simulink model "MPC_RL_H2DF"  (R2023a)
settings: Solver=FixedStepAuto  StartTime=0.0  StopTime=inf  FixedStep=Ts  RelTol=1e-3
model workspace (MAT data in the model file):
  enable_IMEP_noise = 100
  enable_IMEP_offset = 1
values from neighbouring files (symbols this model uses):
  C2C_NMPC = init_C2C_NMPC_H2DF(C2C_NMPC.expdata)    [init_H2DFRL_GRU.m]
  LowerLimit = ([0.17e-3;350;-5;1e-3] - C2C_NMPC.Normalization.controls.mean)./(C2C_NMPC.Normalization.controls.std)    [init_H2DFRL_GRU.m]
  Ts = 0.08    [init_H2DFRL_GRU.m]
  UpperLimit = ([0.5e-3;900;2;5.5e-3] - C2C_NMPC.Normalization.controls.mean)./(C2C_NMPC.Normalization.controls.std)    [init_H2DFRL_GRU.m]
undefined symbols (not defined in the file or in its folder): CA50_offset, DiscIntNeverNeededParam, enable_CA50_noise, enable_CA50_offset, IMEP_offset
libraries: simulink x15, matrix_library x6, dspsigattribs x2, slctrlblks x2, statsLibrary x1, rllib x1
(part 1 of 4)
settings Model: Creator=norouziy  LastModifiedBy=vasu3
settings DebuggingCC: ParameterPrecisionLossMsg=none  UnconnectedInputMsg=warning  UnconnectedOutputMsg=warning  UnconnectedLineMsg=warning
settings ModelReferenceCC: EnableRefExpFcnMdlSchedulingChecks=on
settings RTWCC: DLArmComputeVersion=19.05

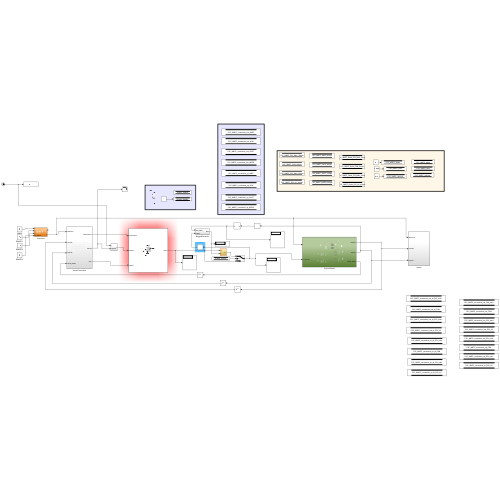
[thumbnail: Simulink's stored preview of the top-level diagram]
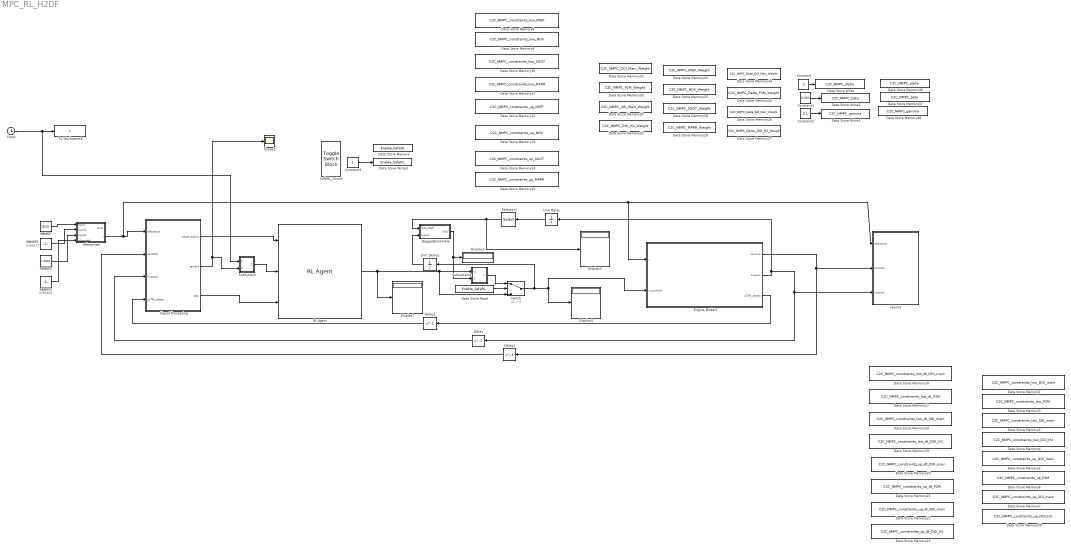
== system MPC_RL_H2DF ==
  BaggedEnsemble : Subsystem
  Clock : Clock
  Constant : Constant  Value=2
  Constant1 : Constant  Value=0.001
  Constant2 : Constant  Value=0.1
  Constant3 : Constant
  Data Store Memory : DataStoreMemory  DataStoreName=Enable_SafeRL  WriteAfterWriteMsg=warning  ShowAdditionalParam=off
  Data Store Memory1 : DataStoreMemory  DataStoreName=C2C_NMPC_constraints_low_DOI_main  WriteAfterWriteMsg=warning  ShowAdditionalParam=off
  Data Store Memory10 : DataStoreMemory  DataStoreName=C2C_NMPC_constraints_low_SOOT  WriteAfterWriteMsg=warning  ShowAdditionalParam=off
  Data Store Memory11 : DataStoreMemory  DataStoreName=C2C_NMPC_constraints_low_MPRR  WriteAfterWriteMsg=warning  ShowAdditionalParam=off
  Data Store Memory12 : DataStoreMemory  DataStoreName=C2C_NMPC_constraints_up_IMEP  WriteAfterWriteMsg=warning  ShowAdditionalParam=off
  Data Store Memory13 : DataStoreMemory  DataStoreName=C2C_NMPC_constraints_up_NOX  WriteAfterWriteMsg=warning  ShowAdditionalParam=off
  Data Store Memory14 : DataStoreMemory  DataStoreName=C2C_NMPC_constraints_up_SOOT  WriteAfterWriteMsg=warning  ShowAdditionalParam=off
  Data Store Memory15 : DataStoreMemory  DataStoreName=C2C_NMPC_constraints_up_MPRR  WriteAfterWriteMsg=warning  ShowAdditionalParam=off
  Data Store Memory16 : DataStoreMemory  DataStoreName=C2C_NMPC_constraints_low_dt_DOI_main  WriteAfterWriteMsg=warning  ShowAdditionalParam=off
  Data Store Memory17 : DataStoreMemory  DataStoreName=C2C_NMPC_constraints_low_dt_P2M  WriteAfterWriteMsg=warning  ShowAdditionalParam=off
  Data Store Memory18 : DataStoreMemory  DataStoreName=C2C_NMPC_constraints_low_dt_SOI_main  WriteAfterWriteMsg=warning  ShowAdditionalParam=off
  Data Store Memory19 : DataStoreMemory  DataStoreName=C2C_NMPC_constraints_low_dt_DOI_H2  WriteAfterWriteMsg=warning  ShowAdditionalParam=off
  Data Store Memory2 : DataStoreMemory  DataStoreName=C2C_NMPC_constraints_low_SOI_main  WriteAfterWriteMsg=warning  ShowAdditionalParam=off
  Data Store Memory20 : DataStoreMemory  DataStoreName=C2C_NMPC_constraints_up_dt_DOI_main  WriteAfterWriteMsg=warning  ShowAdditionalParam=off
  Data Store Memory21 : DataStoreMemory  DataStoreName=C2C_NMPC_constraints_up_dt_P2M  WriteAfterWriteMsg=warning  ShowAdditionalParam=off
  Data Store Memory22 : DataStoreMemory  DataStoreName=C2C_NMPC_constraints_up_dt_SOI_main  WriteAfterWriteMsg=warning  ShowAdditionalParam=off
  Data Store Memory23 : DataStoreMemory  DataStoreName=C2C_NMPC_constraints_up_dt_DOI_H1  WriteAfterWriteMsg=warning  ShowAdditionalParam=off
  Data Store Memory24 : DataStoreMemory  DataStoreName=C2C_NMPC_IMEP_Weight  WriteAfterWriteMsg=warning  ShowAdditionalParam=off
  Data Store Memory25 : DataStoreMemory  DataStoreName=C2C_NMPC_NOX_Weight  WriteAfterWriteMsg=warning  ShowAdditionalParam=off
  Data Store Memory26 : DataStoreMemory  DataStoreName=C2C_NMPC_Delta_SOI_Main_Weight  WriteAfterWriteMsg=warning  ShowAdditionalParam=off
  Data Store Memory27 : DataStoreMemory  DataStoreName=C2C_NMPC_Delta_DOI_H2_Weight  WriteAfterWriteMsg=warning  ShowAdditionalParam=off
  Data Store Memory28 : DataStoreMemory  DataStoreName=C2C_NMPC_SOOT_Weight  WriteAfterWriteMsg=warning  ShowAdditionalParam=off
  Data Store Memory29 : DataStoreMemory  DataStoreName=C2C_NMPC_MPRR_Weight  WriteAfterWriteMsg=warning  ShowAdditionalParam=off
  Data Store Memory3 : DataStoreMemory  DataStoreName=C2C_NMPC_constraints_low_P2M  WriteAfterWriteMsg=warning  ShowAdditionalParam=off
  Data Store Memory30 : DataStoreMemory  DataStoreName=C2C_NMPC_SOI_Main_Weight  WriteAfterWriteMsg=warning  ShowAdditionalParam=off
  Data Store Memory31 : DataStoreMemory  DataStoreName=C2C_NMPC_DOI_H2_Weight  WriteAfterWriteMsg=warning  ShowAdditionalParam=off
  Data Store Memory32 : DataStoreMemory  DataStoreName=C2C_NMPC_DOI_Main_Weight  WriteAfterWriteMsg=warning  ShowAdditionalParam=off
  Data Store Memory33 : DataStoreMemory  DataStoreName=C2C_NMPC_P2M_Weight  WriteAfterWriteMsg=warning  ShowAdditionalParam=off
  Data Store Memory34 : DataStoreMemory  DataStoreName=C2C_NMPC_Delta_DOI_Main_Weight  WriteAfterWriteMsg=warning  ShowAdditionalParam=off
  Data Store Memory35 : DataStoreMemory  DataStoreName=C2C_NMPC_Delta_P2M_Weight  WriteAfterWriteMsg=warning  ShowAdditionalParam=off
  Data Store Memory36 : DataStoreMemory  DataStoreName=C2C_NMPC_alpha  WriteAfterWriteMsg=warning  ShowAdditionalParam=off
  Data Store Memory37 : DataStoreMemory  DataStoreName=C2C_NMPC_beta  WriteAfterWriteMsg=warning  ShowAdditionalParam=off
  Data Store Memory38 : DataStoreMemory  DataStoreName=C2C_NMPC_gamma  WriteAfterWriteMsg=warning  ShowAdditionalParam=off
  Data Store Memory39 : DataStoreMemory  DataStoreName=C2C_NMPC_constraints_up_DOI_H2  WriteAfterWriteMsg=warning  ShowAdditionalParam=off
  Data Store Memory4 : DataStoreMemory  DataStoreName=C2C_NMPC_constraints_low_DOI_H2  WriteAfterWriteMsg=warning  ShowAdditionalParam=off
  Data Store Memory5 : DataStoreMemory  DataStoreName=C2C_NMPC_constraints_up_DOI_main  WriteAfterWriteMsg=warning  ShowAdditionalParam=off
  Data Store Memory6 : DataStoreMemory  DataStoreName=C2C_NMPC_constraints_up_P2M  WriteAfterWriteMsg=warning  ShowAdditionalParam=off
  Data Store Memory7 : DataStoreMemory  DataStoreName=C2C_NMPC_constraints_up_SOI_main  WriteAfterWriteMsg=warning  ShowAdditionalParam=off
  Data Store Memory8 : DataStoreMemory  DataStoreName=C2C_NMPC_constraints_low_IMEP  WriteAfterWriteMsg=warning  ShowAdditionalParam=off
  Data Store Memory9 : DataStoreMemory  DataStoreName=C2C_NMPC_constraints_low_NOX  WriteAfterWriteMsg=warning  ShowAdditionalParam=off
  Data Store Read : DataStoreRead  DataStoreName=Enable_SafeRL  IndexOptions=Index vector (dialog)  Indices=1  OutputSizes=1
  Data Store Write : DataStoreWrite  DataStoreName=C2C_NMPC_alpha  IndexOptions=Index vector (dialog)  Indices=1  OutputSizes=1
  Data Store Write1 : DataStoreWrite  DataStoreName=C2C_NMPC_beta  IndexOptions=Index vector (dialog)  Indices=1  OutputSizes=1
  Data Store Write2 : DataStoreWrite  DataStoreName=C2C_NMPC_gamma  IndexOptions=Index vector (dialog)  Indices=1  OutputSizes=1
  Data Store Write3 : DataStoreWrite  DataStoreName=Enable_SafeRL  IndexOptions=Index vector (dialog)  Indices=1  OutputSizes=1
  Delay : Delay  DelayLength=1  InitialCondition=rand(size(C2C_NMPC.xu0))
  Delay1 : Delay  DelayLength=1  InitialCondition=rand(8,1)
  Delay2 : Delay  DelayLength=1  InitialCondition=rand(size(C2C_NMPC.xu0))
  Display{1..4} (4 alike) : Display
  Engine Model2 : Subsystem
  RBMEP : Constant  Value=350220
  RBMEP1 : Constant  Value=0.56473
  RBMEP2 : Constant  Value=1.2601
  RBMEP3 : Constant  Value=0.95402
  RL Agent : rllib/RL Agent  Agent=saved_agent  ExternalActionAsInput=off  ProvideLastAction=off  ProvideCumRwd=off  TreatAsDirectFeedthrough=on  UseStrictObservationDataTypes=off
  SafeRL_Switch : ToggleSwitchBlock
      settings: Values={{'Off', 'On'}, [0 1]}
  Scope1 : Scope
  Selector1 : Selector  IndexOptions=Index vector (dialog)  Indices=[1]  OutputSizes=1
  Signal Processing : Subsystem
  Subsystem : Subsystem
  Subsystem1 : Subsystem
  Switch : Switch  Criteria=u2 > Threshold  SaturateOnIntegerOverflow=off  InputSameDT=off
  To Workspace8 : ToWorkspace  VariableName=t  SaveFormat=Timeseries  SampleTime=-1
  Unit Delay : UnitDelay  SampleTime=-1  HasFrameUpgradeWarning=on
  Unit Delay1 : UnitDelay  SampleTime=-1  HasFrameUpgradeWarning=on
  references : Subsystem
  results : Subsystem
  wires:
  Clock/1 -> Subsystem/1(In1), To Workspace8/1
  Signal Processing/2(reward) -> Scope1/1, Subsystem/2(reward)
  Signal Processing/3(stop) -> RL Agent/3
  Signal Processing/1(observations) -> RL Agent/1
  RBMEP/1 -> references/1(Input)
  references/2(r) -> Engine Model2/1(r), results/1(reference), Signal Processing/1(reference)
  Delay/1 -> Signal Processing/3(Outputs)
  Constant2/1 -> Data Store Write2/1
  Constant1/1 -> Data Store Write1/1
  Constant/1 -> Data Store Write/1
  Delay1/1 -> Signal Processing/4(LSTM_states)
  RBMEP1/1 -> references/2(Input1)
  RBMEP2/1 -> references/3(Input2)
  Subsystem/1(Out1) -> RL Agent/2
  Delay2/1 -> Signal Processing/2(controls)
  Engine Model2/1(controls) -> Delay2/1, results/2(controls)
  Engine Model2/2(outputs) -> Unit Delay/1, Delay/1, results/3(outputs)
  Engine Model2/3(LSTM_states) -> Delay1/1
  BaggedEnsemble/1(NOx) -> Subsystem1/2(In1), Display2/1
  RL Agent/1 -> Subsystem1/1(u1), Switch/3, Display1/1
  Unit Delay/1 -> Selector1/1
  Selector1/1 -> BaggedEnsemble/1(last_IMEP), Display3/1
  Subsystem1/1(u*1) -> Switch/1
  RBMEP3/1 -> references/4(rchange4)
  Data Store Read/1 -> Switch/2
  Switch/1 -> Unit Delay1/1, Engine Model2/2(rl_controls), Display4/1
  Constant3/1 -> Data Store Write3/1
  Unit Delay1/1 -> BaggedEnsemble/2(Inputs)

== system MPC_RL_H2DF/BaggedEnsemble ==
  last_IMEP : Inport
  Inputs : Inport  Port=2
  Mux : Mux  Inputs=2
  RegressionEnsemble Predict : statsLibrary/Regression/RegressionEnsemble Predict  TrainedLearner=trainedModel.RegressionEnsemble  OutMin=[]  OutMax=[]  WeakLearnerOutMin=[]  WeakLearnerOutMax=[]
  NOx : Outport
  wires:
  Mux/1 -> RegressionEnsemble Predict/1
  RegressionEnsemble Predict/1 -> NOx/1
  Inputs/1 -> Mux/1
  last_IMEP/1 -> Mux/2

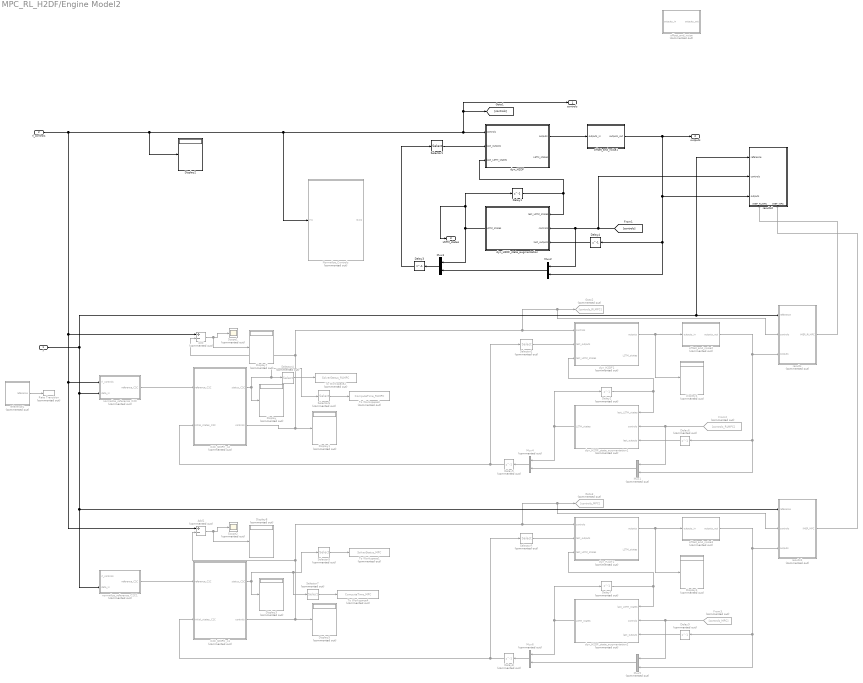
== system MPC_RL_H2DF/Engine Model2 ==
  r : Inport
  rl_controls : Inport  Port=2
  Add : Sum  Commented=on  Inputs=+-
  Add1 : Sum  Commented=on  Inputs=+-
  C2C_NMPC_n1 : Subsystem  Commented=on  VariantControl=C2C_NMPC_n2
  C2C_NMPC_n2 : Subsystem  Commented=on  VariantControl=C2C_NMPC_n2
  Delay1 : Delay  DelayLength=1  InitialCondition=C2C_NMPC.x0(1:C2C_NMPC.Dims.n_LSTM_states)
  Delay2 : Delay  Commented=on  DelayLength=1  InitialCondition=C2C_NMPC.x0(1:C2C_NMPC.Dims.n_LSTM_states)
  Delay3 : Delay  DelayLength=1  InitialCondition=C2C_NMPC.x0
  Delay4 : Delay  DelayLength=1  InitialCondition=C2C_NMPC.x0((C2C_NMPC.Dims.n_states - C2C_NMPC.Dims.n_outputs + 1):C2C_NMPC.Dims.n_states)
  Delay5 : Delay  Commented=on  DelayLength=1  InitialCondition=C2C_NMPC.x0
  Delay6 : Delay  Commented=on  DelayLength=1  InitialCondition=C2C_NMPC.x0((C2C_NMPC.Dims.n_states - C2C_NMPC.Dims.n_outputs + 1):C2C_NMPC.Dims.n_states)
  Delay7 : Delay  Commented=on  DelayLength=1  InitialCondition=C2C_NMPC.x0(1:C2C_NMPC.Dims.n_LSTM_states)
  Delay8 : Delay  Commented=on  DelayLength=1  InitialCondition=C2C_NMPC.x0
  Delay9 : Delay  Commented=on  DelayLength=1  InitialCondition=C2C_NMPC.x0((C2C_NMPC.Dims.n_states - C2C_NMPC.Dims.n_outputs + 1):C2C_NMPC.Dims.n_states)
  Display{,1,3..8} (8 alike) : Display  Commented=on
  Display2 : Display
  From2 : From  Commented=on  GotoTag=controls_RLMPC
  From3 : From  Commented=on  GotoTag=controls_MPC
  Goto2 : Goto  Commented=on  GotoTag=controls_RLMPC
  Goto3 : Goto  Commented=on  GotoTag=controls_MPC
  Mux{1,4..6} (4 alike) : Mux  Commented=on  Inputs=2
  Mux2 : Mux  Inputs=2
  Mux3 : Mux  Inputs=2
  Normalise_Controls : Subsystem  Commented=on
  Rate Transition : RateTransition  Commented=on  Integrity=off  OutPortSampleTime=Ts
  Scope1 : Scope  Commented=on
  Scope2 : Scope  Commented=on
  Selector1 : Selector  IndexOptions=Index vector (dialog)  Indices=[(C2C_NMPC.Dims.n_states - C2C_NMPC.Dims.n_outputs + 1):C2C_NMPC.Dims.n_states]  OutputSizes=1
  Selector2 : Selector  Commented=on  IndexOptions=Index vector (dialog)  Indices=[(C2C_NMPC.Dims.n_states - C2C_NMPC.Dims.n_outputs + 1):C2C_NMPC.Dims.n_states]  OutputSizes=1
  Selector3 : Selector  Commented=on  IndexOptions=Index vector (dialog)  Indices=[(C2C_NMPC.Dims.n_states - C2C_NMPC.Dims.n_outputs + 1):C2C_NMPC.Dims.n_states]  OutputSizes=1
  Selector4 : Selector  Commented=on  IndexOptions=Index vector (dialog)  Indices=1  OutputSizes=1
  Selector5 : Selector  Commented=on  IndexOptions=Index vector (dialog)  Indices=1  OutputSizes=1
  Selector6 : Selector  Commented=on  IndexOptions=Index vector (dialog)  Indices=3  OutputSizes=1
  Selector7 : Selector  Commented=on  IndexOptions=Index vector (dialog)  Indices=3  OutputSizes=1
  To Workspace1 : ToWorkspace  Commented=on  VariableName=SolverStatus_MPC  SampleTime=-1
  To Workspace2 : ToWorkspace  Commented=on  VariableName=SolverStatus_RLMPC  SampleTime=-1
  To Workspace3 : ToWorkspace  Commented=on  VariableName=ComputeTime_RLMPC  SampleTime=-1
  To Workspace4 : ToWorkspace  Commented=on  VariableName=ComputeTime_MPC  SampleTime=-1
  dyn_H2DF : Subsystem
  dyn_H2DF1 : Subsystem  Commented=on
  dyn_H2DF2 : Subsystem  Commented=on
  dyn_H2DF_state_augmentation : Subsystem
  dyn_H2DF_state_augmentation1 : Subsystem  Commented=on
  dyn_H2DF_state_augmentation2 : Subsystem  Commented=on
  normalize_reference_C2C : Subsystem  Commented=on
  normalize_reference_C2C1 : Subsystem  Commented=on
  offset_and_noise : Subsystem  Commented=on
  offset_and_noise1 : Subsystem
  offset_and_noise2 : Subsystem  Commented=on
  offset_and_noise3 : Subsystem  Commented=on
  reference1 : Subsystem  Commented=on
  results : Subsystem  Commented=on
  results1 : Subsystem  Commented=on
  results2 : Subsystem
      settings: PortSchema="{\"entries\":[{\"content\":{\"sides\":[{\"content\":{\"connectorIds\":[\"In1\",\"In2\",\"In3\"]},\"type\":\"ConnectorPlacement.EquallySpacedRectSide\",\"uuid\":\"75c69b80-8417-4b18-a9f8-39f8bddf459c\"},{\"content\":{\"side\":\"RIGHT\"},\"type\":\"ConnectorPlacement.EquallySpacedRectSide\",\"uuid\":\"4217b16a-0e70-4cec-a2f5-17ebe6dd1f5c\"},{\"content\":{\"side\":\"TOP\"},\"type\":\"ConnectorPlacement.EquallySpacedRectSide\",\"uuid\":\"1a4bc296-7285-4f1a-9d1a-4ffa534b2784\"},{\"content\":{\"connectorIds\":[\"In4\",\"In5\"],\"side\":\"BOTTOM\"},\"type\":\"ConnectorPlacement.EquallySpacedRectSide\",\"uuid\":\"31d565b7-d93d-4aac-b998-bcfa263f4420\"}]},\"type\":\"ConnectorPlacement.EquallySpacedConnector\",\"uuid\":\"a3bd06e2-48d8-47a5-9635-2e0335e011af\"}],\"packageUris\":[\"http://schema.mathworks.com/mf0/Connector/R2020b\"],\"version\":\"1.0\"}"
  controls : Outport
  outputs : Outport  Port=2
  LSTM_states : Outport  Port=3
  wires:
  Mux3/1 -> Delay3/1
  Delay1/1 -> dyn_H2DF/3(last_LSTM_states), dyn_H2DF_state_augmentation/1(last_LSTM_states)
  [controls] -> results2/2(controls), dyn_H2DF_state_augmentation/2(controls), Mux2/1
  Delay3/1 -> Selector1/1
  Delay4/1 -> dyn_H2DF_state_augmentation/3(last_outputs)
  Mux2/1 -> Mux3/2
  Selector1/1 -> dyn_H2DF/2(last_outputs)
  dyn_H2DF/1(outputs) -> offset_and_noise1/1(outputs_in)
  dyn_H2DF_state_augmentation/1(LSTM_states) -> LSTM_states/1, Delay1/1, Mux3/1
  offset_and_noise1/1(outputs_out) -> results2/3(outputs), Delay4/1, Mux2/2, outputs/1
  normalize_reference_C2C/1(reference_C2C) -> C2C_NMPC_n2/1(reference_C2C)
  C2C_NMPC_n2/2(controls) -> Add/2, results/2(controls), Goto2/1, dyn_H2DF1/1(controls), Display1/1
  reference1/1(reference) -> Rate Transition/1
  Delay6/1 -> dyn_H2DF_state_augmentation1/3(last_outputs)
  C2C_NMPC_n2/1(status_C2C) -> Selector6/1, Selector4/1, Display/1
  Mux1/1 -> Mux4/2
  dyn_H2DF_state_augmentation1/1(LSTM_states) -> Delay2/1, Mux4/1
  From2/1 -> dyn_H2DF_state_augmentation1/2(controls), Mux1/1
  dyn_H2DF1/1(outputs) -> Display4/1, offset_and_noise2/1(outputs_in)
  Mux4/1 -> Delay5/1
  Selector2/1 -> dyn_H2DF1/2(last_outputs)
  Delay5/1 -> C2C_NMPC_n2/2(initial_states_C2C), Selector2/1
  Delay2/1 -> dyn_H2DF1/3(last_LSTM_states), dyn_H2DF_state_augmentation1/1(last_LSTM_states)
  Add/1 -> Display7/1, Scope1/1
  offset_and_noise2/1(outputs_out) -> results/3(outputs), Delay6/1, Mux1/2
  normalize_reference_C2C1/1(reference_C2C) -> C2C_NMPC_n1/1(reference_C2C)
  Mux5/1 -> Mux6/2
  Mux6/1 -> Delay8/1
  dyn_H2DF2/1(outputs) -> Display6/1, offset_and_noise3/1(outputs_in)
  From3/1 -> dyn_H2DF_state_augmentation2/2(controls), Mux5/1
  offset_and_noise3/1(outputs_out) -> results1/3(outputs), Delay9/1, Mux5/2
  C2C_NMPC_n1/2(controls) -> results1/2(controls), Goto3/1, dyn_H2DF2/1(controls), Add1/2, Display5/1
  Delay7/1 -> dyn_H2DF2/3(last_LSTM_states), dyn_H2DF_state_augmentation2/1(last_LSTM_states)
  Add1/1 -> Display8/1, Scope2/1
  Delay9/1 -> dyn_H2DF_state_augmentation2/3(last_outputs)
  Delay8/1 -> C2C_NMPC_n1/2(initial_states_C2C), Selector3/1
  Selector3/1 -> dyn_H2DF2/2(last_outputs)
  dyn_H2DF_state_augmentation2/1(LSTM_states) -> Delay7/1, Mux6/1
  rl_controls/1 -> Display2/1, Normalise_Controls/1(In1), controls/1, [controls], dyn_H2DF/1(controls), Add1/1, normalize_reference_C2C/1(rl_controls), Add/1
  r/1 -> results1/1(reference), normalize_reference_C2C1/2(data_in), normalize_reference_C2C/2(data_in), results2/1(reference), results/1(reference)
  results/1(IMEP_RLMPC) -> results2/4(IMEP_RLMPC)
  results1/1(IMEP_MPC) -> results2/5(IMEP_MPC)
  Selector4/1 -> To Workspace2/1
  Selector5/1 -> To Workspace1/1
  Selector6/1 -> To Workspace3/1
  Selector7/1 -> To Workspace4/1
  C2C_NMPC_n1/1(status_C2C) -> Display3/1, Selector7/1, Selector5/1

== system MPC_RL_H2DF/Signal Processing ==
  reference : Inport
  controls : Inport  Port=2
  Outputs : Inport  Port=3
  LSTM_states : Inport  Port=4
  Normalization : Subsystem  Commented=on
  calculate reward : Subsystem
  generate observations1 : Subsystem
  stop simulation : Subsystem
  observations : Outport
  reward : Outport  Port=2
  stop : Outport  Port=3
  wires:
  calculate reward/1(reward) -> reward/1
  stop simulation/1(stop) -> stop/1
  generate observations1/1(observations) -> observations/1
  reference/1 -> generate observations1/2(Reference), calculate reward/1(Reference)
  Outputs/1 -> stop simulation/1(Output), calculate reward/3(outputs), generate observations1/1(Outputs)
  controls/1 -> calculate reward/2(controls)
  LSTM_states/1 -> generate observations1/3(LSTM States)

== system MPC_RL_H2DF/Subsystem ==
  In1 : Inport
  reward : Inport  Port=2
  If : If  IfExpression=u1 > 0.08
  If Action Subsystem : Subsystem  TreatAsAtomicUnit=on
  If Action Subsystem1 : Subsystem  TreatAsAtomicUnit=on
  Merge : Merge
  Out1 : Outport
  wires:
  If/1 -> If Action Subsystem/Action
  If/2 -> If Action Subsystem1/Action
  If Action Subsystem1/1(Out1) -> Merge/2
  If Action Subsystem/1(Out1) -> Merge/1
  reward/1 -> If Action Subsystem/1(In1)
  In1/1 -> If/1
  Merge/1 -> Out1/1

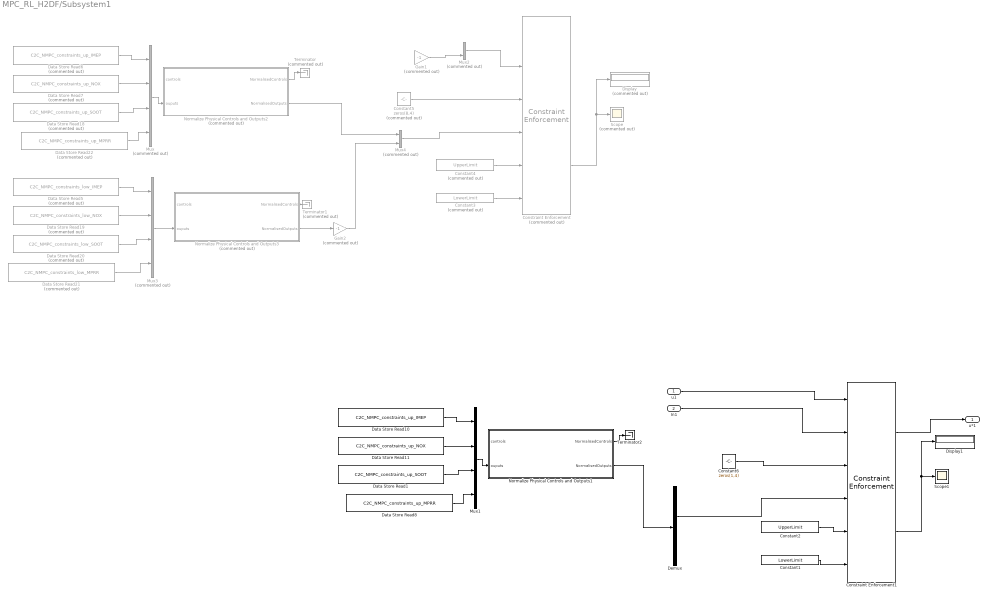
== system MPC_RL_H2DF/Subsystem1 ==
  u1 : Inport
  In1 : Inport  Port=2
  Constant1 : Constant  Value=LowerLimit
  Constant2 : Constant  Value=UpperLimit
  Constant3 : Constant  Commented=on  Value=LowerLimit
  Constant4 : Constant  Commented=on  Value=UpperLimit
  Constant5 : Constant  Commented=on  Value=zeros(8,4)
  Constant6 : Constant  Value=zeros(1,4)
  Constraint Enforcement : slctrlblks/Constraint Enforcement  Commented=on  nc=8  nu=4  c=-0.14  external_c=on  external_umax=on  external_umin=on  Ts=0.08  maxiter=400  tol=1e-6  output_exitflag=on  relax_c=off  relax_u=off
  Constraint Enforcement1 : slctrlblks/Constraint Enforcement  nc=1  nu=4  c=-0.14  external_c=on  external_umax=on  external_umin=on  Ts=Ts  maxiter=400  tol=1e-6  output_exitflag=on  relax_c=off  relax_u=off
  Data Store Read1 : DataStoreRead  DataStoreName=C2C_NMPC_constraints_up_SOOT  IndexOptions=Index vector (dialog)  Indices=1  OutputSizes=1
  Data Store Read10 : DataStoreRead  DataStoreName=C2C_NMPC_constraints_up_IMEP  IndexOptions=Index vector (dialog)  Indices=1  OutputSizes=1
  Data Store Read11 : DataStoreRead  DataStoreName=C2C_NMPC_constraints_up_NOX  IndexOptions=Index vector (dialog)  Indices=1  OutputSizes=1
  Data Store Read18 : DataStoreRead  Commented=on  DataStoreName=C2C_NMPC_constraints_up_SOOT  IndexOptions=Index vector (dialog)  Indices=1  OutputSizes=1
  Data Store Read19 : DataStoreRead  Commented=on  DataStoreName=C2C_NMPC_constraints_low_NOX  IndexOptions=Index vector (dialog)  Indices=1  OutputSizes=1
  Data Store Read20 : DataStoreRead  Commented=on  DataStoreName=C2C_NMPC_constraints_low_SOOT  IndexOptions=Index vector (dialog)  Indices=1  OutputSizes=1
  Data Store Read21 : DataStoreRead  Commented=on  DataStoreName=C2C_NMPC_constraints_low_MPRR  IndexOptions=Index vector (dialog)  Indices=1  OutputSizes=1
  Data Store Read22 : DataStoreRead  Commented=on  DataStoreName=C2C_NMPC_constraints_up_MPRR  IndexOptions=Index vector (dialog)  Indices=1  OutputSizes=1
  Data Store Read5 : DataStoreRead  Commented=on  DataStoreName=C2C_NMPC_constraints_low_IMEP  IndexOptions=Index vector (dialog)  Indices=1  OutputSizes=1
  Data Store Read6 : DataStoreRead  Commented=on  DataStoreName=C2C_NMPC_constraints_up_IMEP  IndexOptions=Index vector (dialog)  Indices=1  OutputSizes=1
  Data Store Read7 : DataStoreRead  Commented=on  DataStoreName=C2C_NMPC_constraints_up_NOX  IndexOptions=Index vector (dialog)  Indices=1  OutputSizes=1
  Data Store Read8 : DataStoreRead  DataStoreName=C2C_NMPC_constraints_up_MPRR  IndexOptions=Index vector (dialog)  Indices=1  OutputSizes=1
  Demux : Demux
  Display : Display  Commented=on
  Display1 : Display
  Gain1 : Gain  Commented=on  Gain=-1
  Gain2 : Gain  Commented=on  Gain=-1
  Mux : Mux  Commented=on
  Mux1 : Mux
  Mux2 : Mux  Commented=on  Inputs=2
  Mux3 : Mux  Commented=on
  Mux4 : Mux  Commented=on  Inputs=2
  Normalize Physical Controls and Outputs1 : Subsystem
  Normalize Physical Controls and Outputs2 : Subsystem  Commented=on
  Normalize Physical Controls and Outputs3 : Subsystem  Commented=on
  Scope : Scope  Commented=on
  Scope1 : Scope
  Terminator : Terminator  Commented=on
  Terminator1 : Terminator  Commented=on
  Terminator2 : Terminator
  u*1 : Outport
  wires:
  Constant3/1 -> Constraint Enforcement/6
  Constant4/1 -> Constraint Enforcement/5
  Constant5/1 -> Constraint Enforcement/3
  Data Store Read18/1 -> Mux/3
  Data Store Read22/1 -> Mux/4
  Normalize Physical Controls and Outputs2/1("NormalisedControls ") -> Terminator/1
  Mux/1 -> Normalize Physical Controls and Outputs2/2("ouputs ")
  Data Store Read6/1 -> Mux/1
  Normalize Physical Controls and Outputs2/2(NormalisedOutputs) -> Mux4/1
  Data Store Read7/1 -> Mux/2
  Constraint Enforcement/2 -> Display/1, Scope/1
  Gain1/1 -> Mux2/2
  Mux2/1 -> Constraint Enforcement/2
  Data Store Read20/1 -> Mux3/3
  Normalize Physical Controls and Outputs3/1("NormalisedControls ") -> Terminator1/1
  Data Store Read21/1 -> Mux3/4
  Data Store Read19/1 -> Mux3/2
  Mux3/1 -> Normalize Physical Controls and Outputs3/2("ouputs ")
  Data Store Read5/1 -> Mux3/1
  Normalize Physical Controls and Outputs3/2(NormalisedOutputs) -> Gain2/1
  Gain2/1 -> Mux4/2
  Mux4/1 -> Constraint Enforcement/4
  Data Store Read10/1 -> Mux1/1
  Constraint Enforcement1/1 -> u*1/1
  Mux1/1 -> Normalize Physical Controls and Outputs1/2("ouputs ")
  Normalize Physical Controls and Outputs1/1("NormalisedControls ") -> Terminator2/1
  Data Store Read8/1 -> Mux1/4
  u1/1 -> Constraint Enforcement1/1
  Data Store Read1/1 -> Mux1/3
  In1/1 -> Constraint Enforcement1/2
  Constant6/1 -> Constraint Enforcement1/3
  Constant1/1 -> Constraint Enforcement1/6
  Constant2/1 -> Constraint Enforcement1/5
  Data Store Read11/1 -> Mux1/2
  Constraint Enforcement1/2 -> Display1/1, Scope1/1
  Normalize Physical Controls and Outputs1/2(NormalisedOutputs) -> Demux/1
  Demux/2 -> Constraint Enforcement1/4

== system MPC_RL_H2DF/references ==
  Input : Inport
  Input1 : Inport  Port=2
  Input2 : Inport  Port=3
  rchange4 : Inport  Port=4
  Clock : Clock
  Display : Display
  MATLAB Function : MATLAB Function  TreatAsAtomicUnit=on
  Mux : Mux  Inputs=2
  Mux1 : Mux  Inputs=2
  Mux2 : Mux
  Mux3 : Mux
  Normalize Reference Controls and Outputs : Subsystem
  Repeating Sequence Stair1 : simulink/Sources/Repeating Sequence Stair  OutValues=0  tsamp=-1  OutMin=[]  OutMax=[]  OutDataTypeStr=double  OutputDataTypeScalingMode=double  OutDataType=fixdt(0,8)  ConRadixGroup=Best Precision: Vector-wise  OutScaling=2^-12
  Reshape : Reshape  OutputDimensionality=Customize  OutputDimensions=[1,9]
  Subsystem1 : Subsystem
  Subsystem4 : Subsystem
  Out1 : Outport
  r : Outport  Port=2
  wires:
  Reshape/1 -> Out1/1
  Mux/1 -> Reshape/1
  Clock/1 -> MATLAB Function/1(t)
  Repeating Sequence Stair1/1 -> Mux/2
  Mux1/1 -> r/1, Display/1, Mux/1
  Input/1 -> MATLAB Function/2(rchange1)
  Input1/1 -> MATLAB Function/3(rchange2)
  Input2/1 -> MATLAB Function/4(rchange3)
  MATLAB Function/1(IMEP_ref) -> Mux2/1
  MATLAB Function/2(NOx_ref) -> Mux2/2
  MATLAB Function/3(SOOT_ref) -> Mux2/3
  MATLAB Function/4(MPRR_ref) -> Mux2/4
  Mux2/1 -> Normalize Reference Controls and Outputs/1("ouputs ")
  MATLAB Function/5(DOI_Main_ref) -> Mux3/1
  MATLAB Function/6(P2M_ref) -> Mux3/2
  MATLAB Function/7(SOI_ref) -> Mux3/3
  MATLAB Function/8(DOI_H2_ref) -> Mux3/4
  Mux3/1 -> Normalize Reference Controls and Outputs/2(controls)
  Normalize Reference Controls and Outputs/1(NormalisedOutputs) -> Mux1/1
  Normalize Reference Controls and Outputs/2("NormalisedControls ") -> Mux1/2
  rchange4/1 -> MATLAB Function/5(rchange4)

== system MPC_RL_H2DF/results ==
  reference : Inport
  controls : Inport  Port=2
  outputs : Inport  Port=3
  Demux{1..4} (4 alike) : Demux
  Mux{1..3,7} (4 alike) : Mux  Inputs=2
  Mux6 : Mux
  Scope : Scope  NumInputPorts=8
  Scope2 : Scope
  Selector5 : Selector  IndexOptions=Index vector (dialog)  Indices=[1:4]  OutputSizes=1
  To Workspace1 : ToWorkspace  VariableName=NOX  SampleTime=-1
  To Workspace2 : ToWorkspace  VariableName=soot  SampleTime=-1
  To Workspace3 : ToWorkspace  VariableName=MPRR  SampleTime=-1
  To Workspace4 : ToWorkspace  VariableName=DOI_main  SampleTime=-1
  To Workspace5 : ToWorkspace  VariableName=SOI_pre  SampleTime=-1
  To Workspace6 : ToWorkspace  VariableName=SOI_main  SampleTime=-1
  To Workspace7 : ToWorkspace  VariableName=DOI_H2  SampleTime=-1
  denormalizing physical controls and outputs : Subsystem
  denormalizing reference : Subsystem
  wires:
  reference/1 -> Selector5/1
  Selector5/1 -> Demux3/1
  outputs/1 -> Demux1/1
  controls/1 -> Demux2/1
  Mux7/1 -> Scope/1
  Mux2/1 -> To Workspace1/1, Scope/2
  Mux3/1 -> To Workspace3/1, Scope/4
  Mux1/1 -> To Workspace2/1, Scope/3
  Demux4/2 -> To Workspace5/1, Scope/6
  Demux4/3 -> To Workspace6/1, Scope/7
  Demux4/1 -> To Workspace4/1, Scope/5
  Mux6/1 -> Demux4/1
  Demux1/1 -> denormalizing physical controls and outputs/1(IMEP_norm)
  Demux1/2 -> denormalizing physical controls and outputs/2(NOX_norm)
  Demux1/3 -> denormalizing physical controls and outputs/3(soot_norm)
  Demux1/4 -> denormalizing physical controls and outputs/4(MPRR_norm)
  Demux2/1 -> denormalizing physical controls and outputs/5(DOI_main_norm)
  Demux2/2 -> denormalizing physical controls and outputs/6(SOI_pre_norm)
  Demux2/3 -> denormalizing physical controls and outputs/7(SOI_main_norm)
  denormalizing physical controls and outputs/1(IMEP) -> Scope2/1, Mux7/2
  denormalizing physical controls and outputs/5(DOI_main) -> Mux6/1
  denormalizing physical controls and outputs/6(SOI_pre) -> Mux6/2
  denormalizing physical controls and outputs/7(SOI_main) -> Mux6/3
  denormalizing physical controls and outputs/2(NOX) -> Mux2/2
  denormalizing physical controls and outputs/3(soot) -> Mux1/2
  denormalizing physical controls and outputs/4(MPRR) -> Mux3/2
  Demux2/4 -> denormalizing physical controls and outputs/8(DOI_H2_norm)
  denormalizing physical controls and outputs/8(DOI_H2) -> Mux6/4
  Demux4/4 -> To Workspace7/1, Scope/8
  Demux3/1 -> denormalizing reference/1(IMEP_norm)
  Demux3/2 -> denormalizing reference/2(NOX_norm)
  Demux3/3 -> denormalizing reference/3(soot_norm)
  Demux3/4 -> denormalizing reference/4(MPRR_norm)
  denormalizing reference/1(IMEP) -> Mux7/1
  denormalizing reference/2(NOX) -> Mux2/1
  denormalizing reference/3(soot) -> Mux1/1
  denormalizing reference/4(MPRR) -> Mux3/1

== system MPC_RL_H2DF/Engine Model2/C2C_NMPC_n1 ==
  note: Note: Usage of Sfunction is as follows:Inputs are:1) lbx_0 - lower bound on x for stage 0, size [24]2) ubx_0 - upper bound on x for stage 0, size [24]3) y_ref_0, size [12]4) y_ref - concatenated for shooting nodes 1 to N-1, size [24]5) y_ref_e, size [8]6) lbx for shooting nodes 1 to N-1, size [8]7) ubx for shooting nodes 1 to N-1, size [8]8) lbx_e (lbx at shooting node N), size [4]9) ubx_e (ubx at shooting node N), size [4]10) lh for shooting nodes 0 to N-1, size [36]11) uh for shooting nodes 0 to N-1, size [36]12) lh_e, size [8]13) uh_e, size [8]14) cost_W in column-major format, that is set for all intermediate shooting nodes: 1 to N-1, size [144]15) cost_W_e in column-major format, size [64]16) reset_solver determines if iterate is set to all zeros before other initializations (x_init, u_init) are set and before solver is called, size [1] Outputs are:1) u0, control input at node 0, size [4]2) utraj, control input concatenated for nodes 0 to N-1, size [12]3) xtraj, state concatenated for nodes 0 to N, size [96]4) acados solver status (0 = SUCCESS)5) cost function value6) KKT residual7) KKT residuals, size [4] (stat, eq, ineq, comp)8) x1, state at node 19) CPU time10) SQP iterations
  reference_C2C : Inport
  initial_states_C2C : Inport  Port=2
  Constant13 : Constant  Value=0
  Constant14 : Constant  Value=4
  Data Type Conversion : DataTypeConversion  SaturateOnIntegerOverflow=off  RndMeth=Floor
  Equal : RelationalOperator  Operator===  OutDataTypeStr=boolean  RndMeth=Simplest  InputSameDT=off
  Mux1 : Mux  Inputs=9
  S-Function : S-Function  FunctionName=acados_solver_sfunction_C2C_NMPC  SFunctionDeploymentMode=off  EnableBusSupport=off
  Selector : Selector  IndexOptions=Index vector (dialog)  Indices=[1:(C2C_NMPC.Dims.n_controls + C2C_NMPC.Dims.n_outputs)]  OutputSizes=1
  Selector1 : Selector  IndexOptions=Index vector (dialog)  Indices=[(C2C_NMPC.Dims.n_LSTM_states + 1):(C2C_NMPC.Dims.n_LSTM_states + C2C_NMPC.Dims.n_controls)]  OutputSizes=1
  Terminator{,1..8} (9 alike) : Terminator
  Unit Delay1 : UnitDelay  SampleTime=-1  HasFrameUpgradeWarning=on
  constraints : Subsystem
  cost_function_weights : Subsystem
  status_C2C : Outport
  controls : Outport  Port=2
  wires:
  S-Function/1 -> Terminator/1
  S-Function/2 -> Mux1/5, Terminator1/1
  S-Function/3 -> Terminator2/1, Mux1/6
  S-Function/4 -> Terminator3/1, Mux1/1, Unit Delay1/1
  S-Function/8 -> Selector1/1, Mux1/9
  S-Function/5 -> Terminator4/1, Mux1/2
  S-Function/6 -> Terminator5/1, Mux1/7
  S-Function/7 -> Terminator6/1, Mux1/8
  S-Function/9 -> Mux1/3, Terminator7/1
  S-Function/10 -> Mux1/4, Terminator8/1
  initial_states_C2C/1 -> S-Function/2, S-Function/1
  reference_C2C/1 -> Selector/1, S-Function/4, S-Function/3
  Selector/1 -> S-Function/5
  Selector1/1 -> controls/1
  Mux1/1 -> status_C2C/1
  constraints/8(ubh_e) -> S-Function/13
  constraints/7(lbh_e) -> S-Function/12
  constraints/6(ubh) -> S-Function/11
  constraints/5(lbh) -> S-Function/10
  constraints/4(ubx_e) -> S-Function/9
  constraints/3(lbx_e) -> S-Function/8
  constraints/2(ubx) -> S-Function/7
  constraints/1(lbx) -> S-Function/6
  Constant14/1 -> Equal/2
  Unit Delay1/1 -> Equal/1
  Equal/1 -> Data Type Conversion/1
  cost_function_weights/1(cost_W) -> S-Function/15, S-Function/14
  Data Type Conversion/1 -> S-Function/17
  cost_function_weights/2(cost_W_e) -> S-Function/16

== system MPC_RL_H2DF/Engine Model2/C2C_NMPC_n2 ==
  note: Note: Usage of Sfunction is as follows:Inputs are:1) lbx_0 - lower bound on x for stage 0, size [24]2) ubx_0 - upper bound on x for stage 0, size [24]3) y_ref_0, size [12]4) y_ref - concatenated for shooting nodes 1 to N-1, size [24]5) y_ref_e, size [8]6) lbx for shooting nodes 1 to N-1, size [8]7) ubx for shooting nodes 1 to N-1, size [8]8) lbx_e (lbx at shooting node N), size [4]9) ubx_e (ubx at shooting node N), size [4]10) lh for shooting nodes 0 to N-1, size [36]11) uh for shooting nodes 0 to N-1, size [36]12) lh_e, size [8]13) uh_e, size [8]14) cost_W in column-major format, that is set for all intermediate shooting nodes: 1 to N-1, size [144]15) cost_W_e in column-major format, size [64]16) reset_solver determines if iterate is set to all zeros before other initializations (x_init, u_init) are set and before solver is called, size [1] Outputs are:1) u0, control input at node 0, size [4]2) utraj, control input concatenated for nodes 0 to N-1, size [12]3) xtraj, state concatenated for nodes 0 to N, size [96]4) acados solver status (0 = SUCCESS)5) cost function value6) KKT residual7) KKT residuals, size [4] (stat, eq, ineq, comp)8) x1, state at node 19) CPU time10) SQP iterations
  reference_C2C : Inport
  initial_states_C2C : Inport  Port=2
  Constant13 : Constant  Value=0
  Constant14 : Constant  Value=4
  Data Type Conversion : DataTypeConversion  SaturateOnIntegerOverflow=off  RndMeth=Floor
  Equal : RelationalOperator  Operator===  OutDataTypeStr=boolean  RndMeth=Simplest  InputSameDT=off
  Mux1 : Mux  Inputs=9
  S-Function : S-Function  FunctionName=acados_solver_sfunction_C2C_NMPC  SFunctionDeploymentMode=off  EnableBusSupport=off
  Selector : Selector  IndexOptions=Index vector (dialog)  Indices=[1:(C2C_NMPC.Dims.n_controls + C2C_NMPC.Dims.n_outputs)]  OutputSizes=1
  Selector1 : Selector  IndexOptions=Index vector (dialog)  Indices=[(C2C_NMPC.Dims.n_LSTM_states + 1):(C2C_NMPC.Dims.n_LSTM_states + C2C_NMPC.Dims.n_controls)]  OutputSizes=1
  Terminator{,1..8} (9 alike) : Terminator
  Unit Delay1 : UnitDelay  SampleTime=-1  HasFrameUpgradeWarning=on
  constraints : Subsystem
  cost_function_weights : Subsystem
  status_C2C : Outport
  controls : Outport  Port=2
  wires:
  S-Function/1 -> Terminator/1
  S-Function/2 -> Mux1/5, Terminator1/1
  S-Function/3 -> Terminator2/1, Mux1/6
  S-Function/4 -> Terminator3/1, Mux1/1, Unit Delay1/1
  S-Function/8 -> Selector1/1, Mux1/9
  S-Function/5 -> Terminator4/1, Mux1/2
  S-Function/6 -> Terminator5/1, Mux1/7
  S-Function/7 -> Terminator6/1, Mux1/8
  S-Function/9 -> Mux1/3, Terminator7/1
  S-Function/10 -> Mux1/4, Terminator8/1
  initial_states_C2C/1 -> S-Function/2, S-Function/1
  reference_C2C/1 -> Selector/1, S-Function/4, S-Function/3
  Selector/1 -> S-Function/5
  Selector1/1 -> controls/1
  Mux1/1 -> status_C2C/1
  constraints/8(ubh_e) -> S-Function/13
  constraints/7(lbh_e) -> S-Function/12
  constraints/6(ubh) -> S-Function/11
  constraints/5(lbh) -> S-Function/10
  constraints/4(ubx_e) -> S-Function/9
  constraints/3(lbx_e) -> S-Function/8
  constraints/2(ubx) -> S-Function/7
  constraints/1(lbx) -> S-Function/6
  Constant14/1 -> Equal/2
  Unit Delay1/1 -> Equal/1
  Equal/1 -> Data Type Conversion/1
  cost_function_weights/1(cost_W) -> S-Function/15, S-Function/14
  Data Type Conversion/1 -> S-Function/17
  cost_function_weights/2(cost_W_e) -> S-Function/16

== system MPC_RL_H2DF/Engine Model2/Normalise_Controls ==
  In1 : Inport
  Constant10 : Constant  Value=C2C_NMPC.Normalization.controls.mean(2)
  Constant11 : Constant  Value=C2C_NMPC.Normalization.controls.mean(3)
  Constant12 : Constant  Value=C2C_NMPC.Normalization.controls.mean(4)
  Constant9 : Constant  Value=C2C_NMPC.Normalization.controls.mean(1)
  Demux1 : Demux
  Gain4 : Gain  Gain=1/C2C_NMPC.Normalization.controls.std(1)
  Gain5 : Gain  Gain=1/C2C_NMPC.Normalization.controls.std(2)
  Gain6 : Gain  Gain=1/C2C_NMPC.Normalization.controls.std(3)
  Gain7 : Gain  Gain=1/C2C_NMPC.Normalization.controls.std(4)
  Mux1 : Mux
  Sum{4,6..8} (4 alike) : Sum  Inputs=|+-
  Out1 : Outport
  wires:
  Sum8/1 -> Gain7/1
  Constant12/1 -> Sum8/2
  Constant11/1 -> Sum7/2
  Demux1/1 -> Sum4/1
  Sum7/1 -> Gain6/1
  Demux1/4 -> Sum8/1
  Gain4/1 -> Mux1/1
  Gain6/1 -> Mux1/3
  Sum6/1 -> Gain5/1
  Gain7/1 -> Mux1/4
  In1/1 -> Demux1/1
  Demux1/2 -> Sum6/1
  Gain5/1 -> Mux1/2
  Demux1/3 -> Sum7/1
  Constant9/1 -> Sum4/2
  Sum4/1 -> Gain4/1
  Constant10/1 -> Sum6/2
  Mux1/1 -> Out1/1

== system MPC_RL_H2DF/Engine Model2/dyn_H2DF ==
  controls : Inport
  last_outputs : Inport  Port=2
  last_LSTM_states : Inport  Port=3
  dyn_H2DF : MATLAB Function  TreatAsAtomicUnit=on
  outputs : Outport
  LSTM_states : Outport  Port=2
  wires:
  dyn_H2DF/1(outputs) -> outputs/1
  controls/1 -> dyn_H2DF/2(controls)
  last_outputs/1 -> dyn_H2DF/3(last_outputs)
  dyn_H2DF/2(LSTM_states) -> LSTM_states/1
  last_LSTM_states/1 -> dyn_H2DF/1(last_LSTM_states)

== system MPC_RL_H2DF/Engine Model2/dyn_H2DF1 ==
  controls : Inport
  last_outputs : Inport  Port=2
  last_LSTM_states : Inport  Port=3
  dyn_H2DF : MATLAB Function  TreatAsAtomicUnit=on
  outputs : Outport
  LSTM_states : Outport  Port=2
  wires:
  dyn_H2DF/1(outputs_MPC) -> outputs/1
  controls/1 -> dyn_H2DF/2(controls_MPC)
  last_outputs/1 -> dyn_H2DF/3(last_outputs_MPC)
  dyn_H2DF/2(LSTM_states_MPC) -> LSTM_states/1
  last_LSTM_states/1 -> dyn_H2DF/1(last_LSTM_states_MPC)

== system MPC_RL_H2DF/Engine Model2/dyn_H2DF2 ==
  controls : Inport
  last_outputs : Inport  Port=2
  last_LSTM_states : Inport  Port=3
  dyn_H2DF : MATLAB Function  TreatAsAtomicUnit=on
  outputs : Outport
  LSTM_states : Outport  Port=2
  wires:
  dyn_H2DF/1(outputs_MPC) -> outputs/1
  controls/1 -> dyn_H2DF/2(controls_MPC)
  last_outputs/1 -> dyn_H2DF/3(last_outputs_MPC)
  dyn_H2DF/2(LSTM_states_MPC) -> LSTM_states/1
  last_LSTM_states/1 -> dyn_H2DF/1(last_LSTM_states_MPC)

== system MPC_RL_H2DF/Engine Model2/dyn_H2DF_state_augmentation ==
  last_LSTM_states : Inport
  controls : Inport  Port=2
  last_outputs : Inport  Port=3
  dyn_H2DF_state_augmentation : MATLAB Function  TreatAsAtomicUnit=on
  LSTM_states : Outport
  wires:
  dyn_H2DF_state_augmentation/1(LSTM_states) -> LSTM_states/1
  last_outputs/1 -> dyn_H2DF_state_augmentation/3(last_outputs)
  last_LSTM_states/1 -> dyn_H2DF_state_augmentation/1(last_LSTM_states)
  controls/1 -> dyn_H2DF_state_augmentation/2(controls)

== system MPC_RL_H2DF/Engine Model2/dyn_H2DF_state_augmentation1 ==
  last_LSTM_states : Inport
  controls : Inport  Port=2
  last_outputs : Inport  Port=3
  dyn_H2DF_state_augmentation : MATLAB Function  TreatAsAtomicUnit=on
  LSTM_states : Outport
  wires:
  dyn_H2DF_state_augmentation/1(LSTM_states) -> LSTM_states/1
  last_outputs/1 -> dyn_H2DF_state_augmentation/3(last_outputs_MPC)
  last_LSTM_states/1 -> dyn_H2DF_state_augmentation/1(last_LSTM_states_MPC)
  controls/1 -> dyn_H2DF_state_augmentation/2(controls_MPC)

== system MPC_RL_H2DF/Engine Model2/dyn_H2DF_state_augmentation2 ==
  last_LSTM_states : Inport
  controls : Inport  Port=2
  last_outputs : Inport  Port=3
  dyn_H2DF_state_augmentation : MATLAB Function  TreatAsAtomicUnit=on
  LSTM_states : Outport
  wires:
  dyn_H2DF_state_augmentation/1(LSTM_states) -> LSTM_states/1
  last_outputs/1 -> dyn_H2DF_state_augmentation/3(last_outputs_MPC)
  last_LSTM_states/1 -> dyn_H2DF_state_augmentation/1(last_LSTM_states_MPC)
  controls/1 -> dyn_H2DF_state_augmentation/2(controls_MPC)

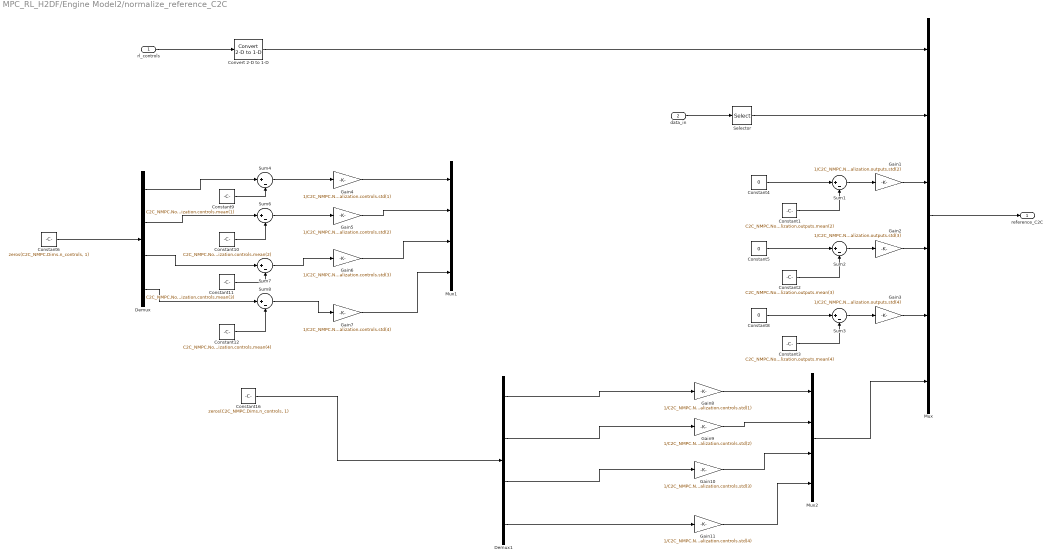
== system MPC_RL_H2DF/Engine Model2/normalize_reference_C2C ==
  rl_controls : Inport
  data_in : Inport  Port=2
  Constant1 : Constant  Value=C2C_NMPC.Normalization.outputs.mean(2)
  Constant10 : Constant  Value=C2C_NMPC.Normalization.controls.mean(2)
  Constant11 : Constant  Value=C2C_NMPC.Normalization.controls.mean(3)
  Constant12 : Constant  Value=C2C_NMPC.Normalization.controls.mean(4)
  Constant16 : Constant  Value=zeros(C2C_NMPC.Dims.n_controls, 1)
  Constant2 : Constant  Value=C2C_NMPC.Normalization.outputs.mean(3)
  Constant3 : Constant  Value=C2C_NMPC.Normalization.outputs.mean(4)
  Constant4 : Constant  Value=0
  Constant5 : Constant  Value=0
  Constant6 : Constant  Value=zeros(C2C_NMPC.Dims.n_controls, 1)
  Constant8 : Constant  Value=0
  Constant9 : Constant  Value=C2C_NMPC.Normalization.controls.mean(1)
  Convert 2-D to 1-D : dspsigattribs/Convert 2-D to 1-D
  Demux : Demux
  Demux1 : Demux
  Gain1 : Gain  Gain=1/C2C_NMPC.Normalization.outputs.std(2)
  Gain10 : Gain  Gain=1/C2C_NMPC.Normalization.controls.std(3)
  Gain11 : Gain  Gain=1/C2C_NMPC.Normalization.controls.std(4)
  Gain2 : Gain  Gain=1/C2C_NMPC.Normalization.outputs.std(3)
  Gain3 : Gain  Gain=1/C2C_NMPC.Normalization.outputs.std(4)
  Gain4 : Gain  Gain=1/C2C_NMPC.Normalization.controls.std(1)
  Gain5 : Gain  Gain=1/C2C_NMPC.Normalization.controls.std(2)
  Gain6 : Gain  Gain=1/C2C_NMPC.Normalization.controls.std(3)
  Gain7 : Gain  Gain=1/C2C_NMPC.Normalization.controls.std(4)
  Gain8 : Gain  Gain=1/C2C_NMPC.Normalization.controls.std(1)
  Gain9 : Gain  Gain=1/C2C_NMPC.Normalization.controls.std(2)
  Mux : Mux  Inputs=6
  Mux1 : Mux
  Mux2 : Mux
  Selector : Selector  IndexOptions=Index vector (dialog)  Indices=1  OutputSizes=1
  Sum{1..4,6..8} (7 alike) : Sum  Inputs=|+-
  reference_C2C : Outport  VectorParamsAs1DForOutWhenUnconnected=off
  wires:
  Mux/1 -> reference_C2C/1
  Gain8/1 -> Mux2/1
  Gain1/1 -> Mux/3
  Demux1/4 -> Gain11/1
  Mux2/1 -> Mux/6
  Demux1/3 -> Gain10/1
  Demux1/1 -> Gain8/1
  Gain9/1 -> Mux2/2
  Demux1/2 -> Gain9/1
  Constant16/1 -> Demux1/1
  Constant1/1 -> Sum1/2
  Sum1/1 -> Gain1/1
  Gain10/1 -> Mux2/3
  Gain11/1 -> Mux2/4
  Constant3/1 -> Sum3/2
  Gain3/1 -> Mux/5
  Constant4/1 -> Sum1/1
  Sum3/1 -> Gain3/1
  Sum2/1 -> Gain2/1
  Constant8/1 -> Sum3/1
  Constant5/1 -> Sum2/1
  Constant2/1 -> Sum2/2
  data_in/1 -> Selector/1
  Gain2/1 -> Mux/4
  rl_controls/1 -> Convert 2-D to 1-D/1
  Convert 2-D to 1-D/1 -> Mux/1
  Constant9/1 -> Sum4/2
  Demux/2 -> Sum6/1
  Sum8/1 -> Gain7/1
  Gain5/1 -> Mux1/2
  Gain7/1 -> Mux1/4
  Demux/4 -> Sum8/1
  Sum4/1 -> Gain4/1
  Demux/1 -> Sum4/1
  Sum7/1 -> Gain6/1
  Sum6/1 -> Gain5/1
  Demux/3 -> Sum7/1
  Constant6/1 -> Demux/1
  Gain6/1 -> Mux1/3
  Constant10/1 -> Sum6/2
  Constant12/1 -> Sum8/2
  Constant11/1 -> Sum7/2
  Gain4/1 -> Mux1/1
  Selector/1 -> Mux/2

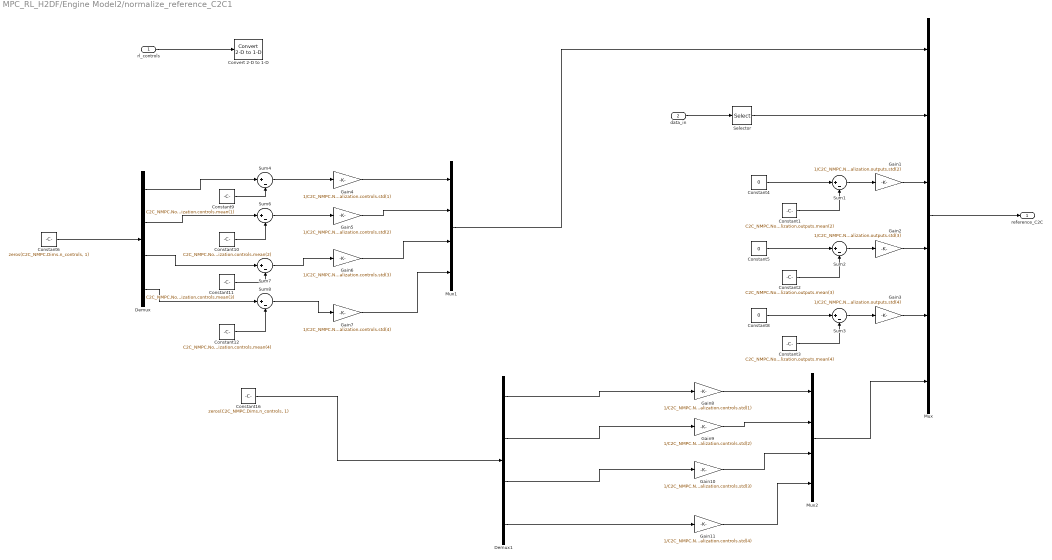
== system MPC_RL_H2DF/Engine Model2/normalize_reference_C2C1 ==
  rl_controls : Inport
  data_in : Inport  Port=2
  Constant1 : Constant  Value=C2C_NMPC.Normalization.outputs.mean(2)
  Constant10 : Constant  Value=C2C_NMPC.Normalization.controls.mean(2)
  Constant11 : Constant  Value=C2C_NMPC.Normalization.controls.mean(3)
  Constant12 : Constant  Value=C2C_NMPC.Normalization.controls.mean(4)
  Constant16 : Constant  Value=zeros(C2C_NMPC.Dims.n_controls, 1)
  Constant2 : Constant  Value=C2C_NMPC.Normalization.outputs.mean(3)
  Constant3 : Constant  Value=C2C_NMPC.Normalization.outputs.mean(4)
  Constant4 : Constant  Value=0
  Constant5 : Constant  Value=0
  Constant6 : Constant  Value=zeros(C2C_NMPC.Dims.n_controls, 1)
  Constant8 : Constant  Value=0
  Constant9 : Constant  Value=C2C_NMPC.Normalization.controls.mean(1)
  Convert 2-D to 1-D : dspsigattribs/Convert 2-D to 1-D
  Demux : Demux
  Demux1 : Demux
  Gain1 : Gain  Gain=1/C2C_NMPC.Normalization.outputs.std(2)
  Gain10 : Gain  Gain=1/C2C_NMPC.Normalization.controls.std(3)
  Gain11 : Gain  Gain=1/C2C_NMPC.Normalization.controls.std(4)
  Gain2 : Gain  Gain=1/C2C_NMPC.Normalization.outputs.std(3)
  Gain3 : Gain  Gain=1/C2C_NMPC.Normalization.outputs.std(4)
  Gain4 : Gain  Gain=1/C2C_NMPC.Normalization.controls.std(1)
  Gain5 : Gain  Gain=1/C2C_NMPC.Normalization.controls.std(2)
  Gain6 : Gain  Gain=1/C2C_NMPC.Normalization.controls.std(3)
  Gain7 : Gain  Gain=1/C2C_NMPC.Normalization.controls.std(4)
  Gain8 : Gain  Gain=1/C2C_NMPC.Normalization.controls.std(1)
  Gain9 : Gain  Gain=1/C2C_NMPC.Normalization.controls.std(2)
  Mux : Mux  Inputs=6
  Mux1 : Mux
  Mux2 : Mux
  Selector : Selector  IndexOptions=Index vector (dialog)  Indices=1  OutputSizes=1
  Sum{1..4,6..8} (7 alike) : Sum  Inputs=|+-
  reference_C2C : Outport  VectorParamsAs1DForOutWhenUnconnected=off
  wires:
  Mux/1 -> reference_C2C/1
  Gain8/1 -> Mux2/1
  Gain1/1 -> Mux/3
  Demux1/4 -> Gain11/1
  Mux2/1 -> Mux/6
  Demux1/3 -> Gain10/1
  Demux1/1 -> Gain8/1
  Gain9/1 -> Mux2/2
  Demux1/2 -> Gain9/1
  Constant16/1 -> Demux1/1
  Constant1/1 -> Sum1/2
  Sum1/1 -> Gain1/1
  Gain10/1 -> Mux2/3
  Gain11/1 -> Mux2/4
  Constant3/1 -> Sum3/2
  Gain3/1 -> Mux/5
  Constant4/1 -> Sum1/1
  Sum3/1 -> Gain3/1
  Sum2/1 -> Gain2/1
  Constant8/1 -> Sum3/1
  Constant5/1 -> Sum2/1
  Constant2/1 -> Sum2/2
  data_in/1 -> Selector/1
  Gain2/1 -> Mux/4
  rl_controls/1 -> Convert 2-D to 1-D/1
  Mux1/1 -> Mux/1
  Constant9/1 -> Sum4/2
  Demux/2 -> Sum6/1
  Sum8/1 -> Gain7/1
  Gain5/1 -> Mux1/2
  Gain7/1 -> Mux1/4
  Demux/4 -> Sum8/1
  Sum4/1 -> Gain4/1
  Demux/1 -> Sum4/1
  Sum7/1 -> Gain6/1
  Sum6/1 -> Gain5/1
  Demux/3 -> Sum7/1
  Constant6/1 -> Demux/1
  Gain6/1 -> Mux1/3
  Constant10/1 -> Sum6/2
  Constant12/1 -> Sum8/2
  Constant11/1 -> Sum7/2
  Gain4/1 -> Mux1/1
  Selector/1 -> Mux/2

== system MPC_RL_H2DF/Engine Model2/offset_and_noise ==
  outputs_in : Inport
  CA50_generation : Subsystem
  IMEP_generation : Subsystem
  Mux : Mux  Inputs=3
  Mux1 : Mux  Inputs=2
  Mux2 : Mux  Inputs=2
  Scope : Scope  NumInputPorts=2
  Selector1 : Selector  IndexOptions=Index vector (dialog)  Indices=[2, 3, 5]  OutputSizes=1
  Selector2 : Selector  IndexOptions=Index vector (dialog)  Indices=[4]  OutputSizes=1
  Selector3 : Selector  IndexOptions=Index vector (dialog)  Indices=[1]  OutputSizes=1
  outputs_out : Outport
  wires:
  Mux/1 -> outputs_out/1
  outputs_in/1 -> Selector3/1, Selector2/1, Selector1/1
  Selector3/1 -> Mux1/2, IMEP_generation/1(IMEP_in)
  Selector1/1 -> Mux/2
  IMEP_generation/1(IMEP_out) -> Mux1/1, Mux/1
  Selector2/1 -> CA50_generation/1(CA50_in), Mux2/2
  CA50_generation/1(CA50_out) -> Mux/3, Mux2/1
  Mux1/1 -> Scope/1
  Mux2/1 -> Scope/2

== system MPC_RL_H2DF/Engine Model2/offset_and_noise1 ==
  outputs_in : Inport
  IMEP_generation : Subsystem
  Mux : Mux  Inputs=2
  Mux1 : Mux  Inputs=2
  Scope : Scope  NumInputPorts=2
  Selector1 : Selector  IndexOptions=Index vector (dialog)  Indices=[2, 3, 4]  OutputSizes=1
  Selector3 : Selector  IndexOptions=Index vector (dialog)  Indices=[1]  OutputSizes=1
  outputs_out : Outport
  wires:
  Mux/1 -> outputs_out/1
  outputs_in/1 -> Selector3/1, Selector1/1
  Selector3/1 -> Mux1/2, Scope/2, IMEP_generation/1(IMEP_in)
  Selector1/1 -> Mux/2
  IMEP_generation/1(IMEP_out) -> Mux1/1, Mux/1
  Mux1/1 -> Scope/1

== system MPC_RL_H2DF/Engine Model2/offset_and_noise2 ==
  outputs_in : Inport
  IMEP_generation : Subsystem
  Mux : Mux  Inputs=2
  Mux1 : Mux  Inputs=2
  Scope : Scope  NumInputPorts=2
  Selector1 : Selector  IndexOptions=Index vector (dialog)  Indices=[2, 3, 4]  OutputSizes=1
  Selector3 : Selector  IndexOptions=Index vector (dialog)  Indices=[1]  OutputSizes=1
  outputs_out : Outport
  wires:
  Mux/1 -> outputs_out/1
  outputs_in/1 -> Selector3/1, Selector1/1
  Selector3/1 -> Mux1/2, Scope/2, IMEP_generation/1(IMEP_in)
  Selector1/1 -> Mux/2
  IMEP_generation/1(IMEP_out) -> Mux1/1, Mux/1
  Mux1/1 -> Scope/1

== system MPC_RL_H2DF/Engine Model2/offset_and_noise3 ==
  outputs_in : Inport
  IMEP_generation : Subsystem
  Mux : Mux  Inputs=2
  Mux1 : Mux  Inputs=2
  Scope : Scope  NumInputPorts=2
  Selector1 : Selector  IndexOptions=Index vector (dialog)  Indices=[2, 3, 4]  OutputSizes=1
  Selector3 : Selector  IndexOptions=Index vector (dialog)  Indices=[1]  OutputSizes=1
  outputs_out : Outport
  wires:
  Mux/1 -> outputs_out/1
  outputs_in/1 -> Selector3/1, Selector1/1
  Selector3/1 -> Mux1/2, Scope/2, IMEP_generation/1(IMEP_in)
  Selector1/1 -> Mux/2
  IMEP_generation/1(IMEP_out) -> Mux1/1, Mux/1
  Mux1/1 -> Scope/1

== system MPC_RL_H2DF/Engine Model2/reference1 ==
  Add1 : Sum  Commented=on
  Clock : Clock  Commented=on
  Constant : Constant  Commented=on
  Constant1 : Constant  Commented=on  Value=C2C_NMPC.ref
  Subsystem4 : Subsystem  Commented=on
  ref_func : MATLAB Function  Commented=on  TreatAsAtomicUnit=on
  reference : Outport  VectorParamsAs1DForOutWhenUnconnected=off
  wires:
  Constant1/1 -> ref_func/1(ref_norm)
  Constant/1 -> Add1/2
  Add1/1 -> ref_func/2(init_index)
  ref_func/1(y_ref) -> reference/1
  Clock/1 -> Add1/1
